simulink model "navigator"  (R2021a)
settings: Solver=FixedStepAuto  StartTime=0.0  StopTime=10.0  FixedStep=0.05  RelTol=1e-3
undefined symbols (not defined in the file): CONSTANTS_RADIUS_OF_EARTH, GF_ACTION, GF_MAX_HOR_DIST, GF_MAX_VER_DIST
(part 2 of 3)

== stateflow chart navigator/Navigator ==
  state navigator
    state COMMAND_SUB [parallel]
      settings: executionOrder=1
      state CMD_DO_GO_AROUND [parallel]
        en:
        % 临时给输出赋值，后续删除
        position_sp_triplet = pos_sp_triplet_input;
        mission_result.timestamp = uint64(getSimulationTime);
        %
        settings: executionOrder=1
        state not_running
        state running
          en:
          %publish_vehicle_command_ack(cmd, vehicle_command_s::VEHICLE_CMD_RESULT_ACCEPTED);
        (default) -> navigator.COMMAND_SUB.CMD_DO_GO_AROUND.not_running
        navigator.COMMAND_SUB.CMD_DO_GO_AROUND.not_running -> navigator.COMMAND_SUB.CMD_DO_GO_AROUND.running : [vehicle_command.command == PX4_VEHICLE_COMMAND.VEHICLE_CMD_DO_GO_AROUND]
        navigator.COMMAND_SUB.CMD_DO_GO_AROUND.running -> navigator.COMMAND_SUB.CMD_DO_GO_AROUND.not_running : [vehicle_command.command ~= PX4_VEHICLE_COMMAND.VEHICLE_CMD_DO_GO_AROUND]
      state CMD_DO_REPOSITION [parallel]
        settings: executionOrder=2
        state not_running
        state running
          en:
          get_reposition_setpoint;
        (default) -> navigator.COMMAND_SUB.CMD_DO_REPOSITION.not_running
        navigator.COMMAND_SUB.CMD_DO_REPOSITION.not_running -> navigator.COMMAND_SUB.CMD_DO_REPOSITION.running : [vehicle_command.command == PX4_VEHICLE_COMMAND.VEHICLE_CMD_DO_REPOSITION ]
        navigator.COMMAND_SUB.CMD_DO_REPOSITION.running -> navigator.COMMAND_SUB.CMD_DO_REPOSITION.not_running : [vehicle_command.command ~= PX4_VEHICLE_COMMAND.VEHICLE_CMD_DO_REPOSITION]
      state CMD_NAV_TAKEOFF [parallel]
        settings: executionOrder=3
        state not_running
        state running
          en:
          % 前一航点
          if ((home_position.timestamp > 0) && home_position.valid_alt && home_position.valid_hpos && home_position.valid_lpos)
          takeoff_triplet_.previous.valid = true;
          takeoff_triplet_.previous.timestamp = uint64(getSimulationTime);
          else
          takeoff_triplet_.previous.valid = false;
          end
          takeoff_triplet_.previous.lat = global_position.lat;
          takeoff_triplet_.previous.lon = global_position.lon;
          takeoff_triplet_.previous.alt = global_position.alt;
          takeoff_triplet_.previous.yaw = local_position.heading;
          % 当前航点
          takeoff_triplet_.current.valid = true;
          takeoff_triplet_.current.timestamp = uint64(getSimulationTime);
          takeoff_triplet_.current.type = uint8(PX4_POSITION_SETPOINT.SETPOINT_TYPE_TAKEOFF);
          if isfinite(vehicle_command.param5) && isfinite(vehicle_command.param6)
          takeoff_triplet_.current.lat = vehicle_command.param5;
          takeoff_triplet_.current.lon = vehicle_command.param6;
          else
          takeoff_triplet_.current.lat = global_position.lat;
          takeoff_triplet_.current.lon = global_position.lon;
          end
          takeoff_triplet_.current.alt = vehicle_command.param7;
          if ((home_position.timestamp > 0) && home_position.valid_alt && home_position.valid_hpos && home_position.valid_lpos)
          takeoff_triplet_.current.yaw = vehicle_command.param4;
          else
          takeoff_triplet_.current.yaw = local_position.heading;
          end
          takeoff_triplet_.current.loiter_radius = NAV_LOITER_RAD;
          takeoff_triplet_.current.loiter_direction = int8(1);
          % 下一航点
          takeoff_triplet_.next.valid = false;
        (default) -> navigator.COMMAND_SUB.CMD_NAV_TAKEOFF.not_running
        navigator.COMMAND_SUB.CMD_NAV_TAKEOFF.not_running -> navigator.COMMAND_SUB.CMD_NAV_TAKEOFF.running : [vehicle_command.command == PX4_VEHICLE_COMMAND.VEHICLE_CMD_NAV_TAKEOFF]
        navigator.COMMAND_SUB.CMD_NAV_TAKEOFF.running -> navigator.COMMAND_SUB.CMD_NAV_TAKEOFF.not_running : [vehicle_command.command ~= PX4_VEHICLE_COMMAND.VEHICLE_CMD_NAV_TAKEOFF]
      state CMD_DO_CHANGE_SPEED [parallel]
        settings: executionOrder=4
        state not_running
        state running
          en,du:
          if (vehicle_command.param2 > eps)
          % 速度指令有效
          if (vehicle_status.vehicle_type == PX4_VEHICLE_STATUS.VEHICLE_TYPE_ROTARY_WING)
          mission_cruising_speed_mc_ = vehicle_command.param2;
          else
          mission_cruising_speed_fw_ = vehicle_command.param2;
          end
          else
          % 速度指令无效
          if (vehicle_status.vehicle_type == PX4_VEHICLE_STATUS.VEHICLE_TYPE_ROTARY_WING)
          mission_cruising_speed_mc_ = single(-1);
          else
          mission_cruising_speed_fw_ = single(-1);
          end
          % 设置油门指令
          if (vehicle_command.param3 > eps)
          mission_throttle_ = vehicle_command.param3 / 100;
          else
          mission_throttle_ = single(nan);
          end
          end
          % TO DO: publish_vehicle_command_ack
        (default) -> navigator.COMMAND_SUB.CMD_DO_CHANGE_SPEED.not_running
        navigator.COMMAND_SUB.CMD_DO_CHANGE_SPEED.not_running -> navigator.COMMAND_SUB.CMD_DO_CHANGE_SPEED.running : [vehicle_command.command==PX4_VEHICLE_COMMAND.VEHICLE_CMD_DO_CHANGE_SPEED]
        navigator.COMMAND_SUB.CMD_DO_CHANGE_SPEED.running -> navigator.COMMAND_SUB.CMD_DO_CHANGE_SPEED.not_running : [vehicle_command.command~=PX4_VEHICLE_COMMAND.VEHICLE_CMD_DO_CHANGE_SPEED]
    state TRAFFIC [parallel]
      settings: executionOrder=2
    state GEOFENCE_CHECK [parallel]
      settings: executionOrder=3
    state SWITCH_NAV_STATE [parallel]
      en,du:
      switch uint8(vehicle_status.nav_state)
      case uint8(PX4_VEHICLE_STATUS.NAVIGATION_STATE_AUTO_MISSION)
      navigation_mode_ = NAVIGATION_MODE.mission;
      case uint8(PX4_VEHICLE_STATUS.NAVIGATION_STATE_AUTO_LOITER)
      navigation_mode_ == NAVIGATION_MODE.loiter;
      case uint8(PX4_VEHICLE_STATUS.NAVIGATION_STATE_AUTO_TAKEOFF)
      navigation_mode_ == NAVIGATION_MODE.takeoff;
      case uint8(PX4_VEHICLE_STATUS.NAVIGATION_STATE_AUTO_LAND)
      navigation_mode_ == NAVIGATION_MODE.land;
      case uint8(PX4_VEHICLE_STATUS.NAVIGATION_STATE_AUTO_LANDENGFAIL)
      navigation_mode_ == NAVIGATION_MODE.engineFailure;
      case uint8(PX4_VEHICLE_STATUS.NAVIGATION_STATE_AUTO_LANDGPSFAIL)
      navigation_mode_ == NAVIGATION_MODE.gpsFailure;
      case uint8(PX4_VEHICLE_STATUS.NAVIGATION_STATE_AUTO_RTL)
      switch RTL_TYPE
      case {int32(PX4_RTL_TYPE.LAND), int32(PX4_RTL_TYPE.CLOSEST)}
      case int32(PX4_RTL_TYPE.MISSION)
      otherwise
      navigation_mode_ = NAVIGATION_MODE.rtl;
      end
      otherwise
      navigation_mode_ = NAVIGATION_MODE.rtl;
      end
      % 记录当前导航状态
      previous_nav_state = vehicle_status.nav_state;
      settings: executionOrder=4
    state NAV_STATE_ACTION [parallel]
      settings: executionOrder=5
      state MISSION [parallel]
        settings: executionOrder=1
        state not_running
        state running
          en:
        (default) -> navigator.NAV_STATE_ACTION.MISSION.not_running
        navigator.NAV_STATE_ACTION.MISSION.not_running -> navigator.NAV_STATE_ACTION.MISSION.running : [navigation_mode_ == NAVIGATION_MODE.mission]
        navigator.NAV_STATE_ACTION.MISSION.running -> navigator.NAV_STATE_ACTION.MISSION.not_running : [navigation_mode_ ~= NAVIGATION_MODE.mission]
      state RTL [parallel]
        settings: executionOrder=2
        state not_running
          en,du:
          rtl_state = PX4_RTL_STATE.NONE;
          find_RTL_destination;
        state running
          en:
          % TO DO: output RTL message, home / mission / safe point
          % 垂起旋翼阶段取消mission方式的降落，因为此处已经不是mission模式了
          deny_mission_landing_ = vehicle_status.is_vtol && (vehicle_status.vehicle_type == PX4_VEHICLE_STATUS.VEHICLE_TYPE_ROTARY_WING);
          get_rtl_alt_and_rad;
          print_des_type;
          state RTL_STATE_CLIMB
            en:
            rtl_state = PX4_RTL_STATE.CLIMB;
            climb_and_return_done_ = false;
            can_loiter_at_sp_ = false;
            % 在当前位置爬升至指定高度
            if (vehicle_status.vehicle_type == PX4_VEHICLE_STATUS.VEHICLE_TYPE_ROTARY_WING)
            % 如果多旋翼则直接爬升到给定高度
            mission_item_.nav_cmd = uint16(PX4_NAVIGATION_CMD.NAV_CMD_WAYPOINT);
            else
            %如果是固定翼，则盘旋上升到给定高度
            mission_item_.nav_cmd = uint16(PX4_NAVIGATION_CMD.NAV_CMD_LOITER_TO_ALT);
            end
            mission_item_.lat = global_position.lat;
            mission_item_.lon = global_position.lon;
            mission_item_.altitude = rtl_alt;
            mission_item_.altitude_is_relative = false;
            mission_item_.yaw = local_position.heading;
            mission_item_.acceptance_radius = navigator.get_acceptance_radius;
            mission_item_.time_inside = single(0);
            mission_item_.autocontinue = true;
            mission_item_.origin =uint8(PX4_MISSION_ORIGIN.ONBOARD);
            sprintf("RTL: climb to %f m (%f m above destination) \t", double(rtl_alt), double(rtl_alt - destination.alt))
            % mavlink_log_info(_navigator->get_mavlink_log_pub(), "RTL: climb to %d m (%d m above destination)\t",(int)ceilf(_rtl_alt), (int)ceilf(_rtl_alt - _destination.alt));
            % Reset all reached flags
            waypoint_position_reached_ = false;
            waypoint_yaw_reached_ = false;
            time_wp_reached_ = uint64(0);
            % TO DO: issue_command
            % 更新当前航点
            mission_item_ = NAV_STATE_ACTION.mission_apply_limitation(mission_item_);
            NAV_STATE_ACTION.mission_item_to_position_setpoint(mission_item_);
            pos_sp_triplet_updated_ = true;
          state RTL_STATE_RETURN
            en:
            rtl_state = PX4_RTL_STATE.RETURN;
            climb_and_return_done_ = false;
            can_loiter_at_sp_ = false;
            % 返航至目标航点
            mission_item_.nav_cmd = uint16(PX4_NAVIGATION_CMD.NAV_CMD_WAYPOINT);
            mission_item_.lat = destination.lat;
            mission_item_.lon = destination.lon;
            mission_item_.altitude = rtl_alt;
            mission_item_.altitude_is_relative = false;
            destination_dist = navigator.get_distance_2_next_waypoint(destination.lat, destination.lon, global_position.lat, global_position.lon);
            if (destination_dist < RTL_MIN_DIST)
            % 如果离着陆点很近，则采用着陆的航向
            mission_item_.yaw = destination.yaw;
            else
            % 否则机头指向着陆点
            mission_item_.yaw = navigator.get_bearing_2_next_waypoint(global_position.lat, global_position.lon, destination.lat, destination.lon);
            end
            mission_item_.acceptance_radius = navigator.get_acceptance_radius;
            mission_item_.time_inside = single(0);
            mission_item_.autocontinue = true;
            mission_item_.origin = uint8(PX4_MISSION_ORIGIN.ONBOARD);
            sprintf("RTL: return at %f m (%f m above destination) \t", double(mission_item_.altitude), double(mission_item_.altitude - destination.alt))
            % Reset all reached flags
            waypoint_position_reached_ = false;
            waypoint_yaw_reached_ = false;
            time_wp_reached_ = uint64(0);
            % TO DO: issue_command
            % 更新当前航点
            mission_item_ = NAV_STATE_ACTION.mission_apply_limitation(mission_item_);
            NAV_STATE_ACTION.mission_item_to_position_setpoint(mission_item_);
            pos_sp_triplet_updated_ = true;
          state RTL_STATE_DESCEND
            en:
            rtl_state = PX4_RTL_STATE.DESCEND;
            climb_and_return_done_ = true;
            can_loiter_at_sp_ = false;
            % 下降至指定高度
            mission_item_.nav_cmd = uint16(PX4_NAVIGATION_CMD.NAV_CMD_LOITER_TO_ALT);
            mission_item_.lat = destination.lat;
            mission_item_.lon = destination.lon;
            mission_item_.altitude = min([destination.alt + RTL_DESCEND_ALT, global_position.alt, rtl_alt]);
            mission_item_.altitude_is_relative = false;
            % Except for vtol which might be still off here and should point towards this location.
            d_current = navigator.get_distance_2_next_waypoint(global_position.lat, global_position.lon, mission_item_.lat, mission_item_.lon);
            if (vehicle_status.is_vtol && (d_current > navigator.get_acceptance_radius))
            mission_item_.yaw = navigator.get_bearing_2_next_waypoint(global_position.lat, global_position.lon, mission_item_.lat, mission_item_.lon);
            else
            mission_item_.yaw = destination.yaw;
            end
            if (vehicle_status.is_vtol)
            mission_item_.loiter_radius = rtl_loiter_rad;
            end
            mission_item_.acceptance_radius = navigator.get_acceptance_radius;
            mission_item_.time_inside = single(0);
            mission_item_.autocontinue = true;
            mission_item_.origin = uint8(PX4_MISSION_ORIGIN.ONBOARD);
            % Disable previous setpoint to prevent drift.
            position_sp_triplet.previous.valid = false;
            sprintf("RTL: descend to %f m (%f m above destination) \t", double(mission_item_.altitude), double(mission_item_.altitude - destination.alt))
            % Reset all reached flags
            waypoint_position_reached_ = false;
            waypoint_yaw_reached_ = false;
            time_wp_reached_ = uint64(0);
            % TO DO: issue_command
            % 更新当前航点
            mission_item_ = NAV_STATE_ACTION.mission_apply_limitation(mission_item_);
            NAV_STATE_ACTION.mission_item_to_position_setpoint(mission_item_);
            pos_sp_triplet_updated_ = true;
          state RTL_STATE_LOITER
            en:
            rtl_state = PX4_RTL_STATE.LOITER;
            climb_and_return_done_ = true;
            can_loiter_at_sp_ = true;
            % Don't change altitude.
            mission_item_.lat = destination.lat;
            mission_item_.lon = destination.lon;
            mission_item_.altitude = min([destination.alt + RTL_DESCEND_ALT, global_position.alt, rtl_alt]);
            mission_item_.altitude_is_relative = false;
            mission_item_.yaw = destination.yaw;
            mission_item_.loiter_radius = NAV_LOITER_RAD;
            mission_item_.acceptance_radius = navigator.get_acceptance_radius;
            mission_item_.time_inside = max(RTL_LAND_DELAY, single(0.0));
            mission_item_.autocontinue = (RTL_LAND_DELAY > eps);
            mission_item_.origin = uint8(PX4_MISSION_ORIGIN.ONBOARD);
            if (RTL_LAND_DELAY > eps)
            mission_item_.nav_cmd = uint16(PX4_NAVIGATION_CMD.NAV_CMD_LOITER_TIME_LIMIT)
            sprintf("RTL: loiter %f. \t", double(mission_item_.time_inside));
            %mavlink_log_info(_navigator->get_mavlink_log_pub(), "RTL: loiter %.1fs\t", (double)get_time_inside(_mission_item));
            %events::send<float>(events::ID("rtl_loiter"), events::Log::Info, "RTL: loiter {1:.1}s", get_time_inside(_mission_item));
            else
            mission_item_.nav_cmd = uint16(PX4_NAVIGATION_CMD.NAV_CMD_LOITER_UNLIMITED);
            sprintf("RTL: completed, loitering. \t")
            %mavlink_log_info(_navigator->get_mavlink_log_pub(), "RTL: completed, loitering\t");
            %events::send(events::ID("rtl_completed_loiter"), events::Log::Info, "RTL: completed, loitering");
            end
            % Reset all reached flags
            waypoint_position_reached_ = false;
            waypoint_yaw_reached_ = false;
            time_wp_reached_ = uint64(0);
            % TO DO: issue_command
            % 更新当前航点
            mission_item_ = NAV_STATE_ACTION.mission_apply_limitation(mission_item_);
            NAV_STATE_ACTION.mission_item_to_position_setpoint(mission_item_);
            pos_sp_triplet_updated_ = true;
          state RTL_STATE_LAND
            en:
            rtl_state = PX4_RTL_STATE.LANDING;
            climb_and_return_done_ = true;
            can_loiter_at_sp_ = false;
            % Land at destination.
            mission_item_.nav_cmd = uint16(PX4_NAVIGATION_CMD.NAV_CMD_LAND);
            mission_item_.lat = destination.lat;
            mission_item_.lon = destination.lon;
            mission_item_.yaw = destination.yaw;
            mission_item_.altitude = destination.alt;
            mission_item_.altitude_is_relative = false;
            mission_item_.acceptance_radius = navigator.get_acceptance_radius;
            mission_item_.time_inside = single(0);
            mission_item_.autocontinue = true;
            mission_item_.origin = uint8(PX4_MISSION_ORIGIN.ONBOARD);
            %mission_item_.land_precision = RTL_PLD_MD;
            %if (mission_item_.land_precision == 1)
            %_navigator->get_precland()->set_mode(PrecLandMode::Opportunistic);
            %_navigator->get_precland()->on_activation();
            %elseif (mission_item_.land_precision == 2)
            %_navigator->get_precland()->set_mode(PrecLandMode::Required);
            %_navigator->get_precland()->on_activation();
            %end
            sprintf("RTL: land at destination")
            %mavlink_log_info(_navigator->get_mavlink_log_pub(), "RTL: land at destination\t");
            % %events::send(events::ID("rtl_land_at_destination"), events::Log::Info, "RTL: land at destination");
            % Reset all reached flags
            waypoint_position_reached_ = false;
            waypoint_yaw_reached_ = false;
            time_wp_reached_ = uint64(0);
            % TO DO: issue_command
            % 更新当前航点
            mission_item_ = NAV_STATE_ACTION.mission_apply_limitation(mission_item_);
            NAV_STATE_ACTION.mission_item_to_position_setpoint(mission_item_);
            pos_sp_triplet_updated_ = true;
          state RTL_MOVE_TO_LAND_HOVER_VTOL
            en:
            rtl_state = PX4_RTL_STATE.MOVE_TO_LAND_HOVER_VTOL;
            climb_and_return_done_ = true;
            can_loiter_at_sp_ = false;
            %
            mission_item_.nav_cmd = uint16(PX4_NAVIGATION_CMD.NAV_CMD_WAYPOINT);
            mission_item_.lat = destination.lat;
            mission_item_.lon = destination.lon;
            mission_item_.altitude = min([destination.alt + RTL_DESCEND_ALT, global_position.alt, rtl_alt]);
            mission_item_.altitude_is_relative = false;
            mission_item_.yaw = navigator.get_bearing_2_next_waypoint(global_position.lat, global_position.lon, mission_item_.lat, mission_item_.lon);
            mission_item_.acceptance_radius = navigator.get_acceptance_radius;
            mission_item_.origin = uint8(PX4_MISSION_ORIGIN.ONBOARD);
            % Reset all reached flags
            waypoint_position_reached_ = false;
            waypoint_yaw_reached_ = false;
            time_wp_reached_ = uint64(0);
            % TO DO: issue_command
            % 更新当前航点
            mission_item_ = NAV_STATE_ACTION.mission_apply_limitation(mission_item_);
            NAV_STATE_ACTION.mission_item_to_position_setpoint(mission_item_);
            pos_sp_triplet_updated_ = true;
          state RTL_STATE_TRANSITION_TO_MC
            en:
            rtl_state = PX4_RTL_STATE.TRANSITION_TO_MC;
            climb_and_return_done_ = true;
            can_loiter_at_sp_ = false;
            % 设置固定翼切换到旋翼的过渡点
            mission_item_.nav_cmd = uint16(PX4_NAVIGATION_CMD.NAV_CMD_DO_VTOL_TRANSITION);
            % params 是union联合体
            mission_item_.time_inside = single(PX4_VTOL_VEHICLE_STATUS.VEHICLE_VTOL_STATE_MC);
            mission_item_.acceptance_radius = single(0.0);
            mission_item_.yaw = local_position.heading;
            mission_item_.autocontinue = true;
            % Reset all reached flags
            waypoint_position_reached_ = false;
            waypoint_yaw_reached_ = false;
            time_wp_reached_ = uint64(0);
            % TO DO: issue_command
            % 更新当前航点
            mission_item_ = NAV_STATE_ACTION.mission_apply_limitation(mission_item_);
            NAV_STATE_ACTION.mission_item_to_position_setpoint(mission_item_);
            pos_sp_triplet_updated_ = true;
          state RTL_STATE_HEAD_TO_CENTER
            en:
            rtl_state = PX4_RTL_STATE.HEAD_TO_CENTER;
            climb_and_return_done_ = true;
            can_loiter_at_sp_ = false;
            %
            mission_item_.nav_cmd = uint16(PX4_NAVIGATION_CMD.NAV_CMD_WAYPOINT);
            mission_item_.lat = destination.lat;
            mission_item_.lon = destination.lon;
            mission_item_.altitude = min([destination.alt + RTL_DESCEND_ALT, global_position.alt, rtl_alt]);
            mission_item_.altitude_is_relative = false;
            mission_item_.yaw = navigator.get_bearing_2_next_waypoint(global_position.lat, global_position.lon, mission_item_.lat, mission_item_.lon);
            mission_item_.acceptance_radius = navigator.get_acceptance_radius;
            mission_item_.time_inside = single(0);
            mission_item_.autocontinue = true;
            mission_item_.origin = uint8(PX4_MISSION_ORIGIN.ONBOARD);
            % Disable previous setpoint to prevent drift.
            position_sp_triplet.previous.valid = false;
            % Reset all reached flags
            waypoint_position_reached_ = false;
            waypoint_yaw_reached_ = false;
            time_wp_reached_ = uint64(0);
            % TO DO: issue_command
            % 更新当前航点
            mission_item_ = NAV_STATE_ACTION.mission_apply_limitation(mission_item_);
            NAV_STATE_ACTION.mission_item_to_position_setpoint(mission_item_);
            pos_sp_triplet_updated_ = true;
          state RTL_STATE_LANDED
            en:
            rtl_state = PX4_RTL_STATE.LANDED
            climb_and_return_done_ = true;
            can_loiter_at_sp_ = false;
            %
            NAV_STATE_ACTION.set_idle_item;
            rtl_alt_min_ = false;
            % Reset all reached flags
            waypoint_position_reached_ = false;
            waypoint_yaw_reached_ = false;
            time_wp_reached_ = uint64(0);
            % TO DO: issue_command
            % 更新当前航点
            mission_item_ = NAV_STATE_ACTION.mission_apply_limitation(mission_item_);
            NAV_STATE_ACTION.mission_item_to_position_setpoint(mission_item_);
            pos_sp_triplet_updated_ = true;
          (default) -> RTL_STATE_DESCEND [order 2] : % 如果rtl降落点类型为MISSION_LANDING，并且飞行器处于正在降落的过程中
              | [destination.type == PX4_RTL_DESTINATION_TYPE.MISSION_LANDING && ...
              | mission_landing_in_progress_]
          (default) -> RTL_STATE_CLIMB [order 3] : % 如果飞行器的高度低于预设的降落高度
              | [global_position.alt < ((destination.alt + RTL_RETURN_ALT) || ...
              | rtl_alt_min_)]
          (default) -> RTL_STATE_RETURN [order 4]
          RTL_STATE_CLIMB -> RTL_STATE_RETURN : [NAV_STATE_ACTION.is_mission_item_reached(mission_item_)]
          RTL_STATE_RETURN -> (junction 800) : [NAV_STATE_ACTION.is_mission_item_reached(mission_item_)]
          (junction 800) -> RTL_STATE_DESCEND [order 1] : [(RTL_LAND_DELAY < -0.01 || RTL_LAND_DELAY > 0.01) || ...
              | (vehicle_status.is_vtol && vehicle_status.vehicle_type == PX4_VEHICLE_STATUS.VEHICLE_TYPE_FIXED_WING)]
          (junction 800) -> (junction 801) [order 2]
          RTL_STATE_DESCEND -> (junction 802) : [NAV_STATE_ACTION.is_mission_item_reached(mission_item_)]
          (junction 802) -> (junction 801) [order 3]
          (junction 802) -> (junction 803) [order 2] : [vehicle_status.is_vtol && ...
              | vehicle_status.vehicle_type == PX4_VEHICLE_STATUS.VEHICLE_TYPE_FIXED_WING]
          (junction 801) -> (junction 805)
          (junction 802) -> RTL_STATE_LOITER [order 1] : [RTL_LAND_DELAY < -0.01 || RTL_LAND_DELAY > 0.01]
          (junction 803) -> RTL_STATE_HEAD_TO_CENTER
          RTL_STATE_LOITER -> (junction 805) : [NAV_STATE_ACTION.is_mission_item_reached(mission_item_)]
          (junction 805) -> (junction 804)
          (junction 804) -> RTL_STATE_LAND
          RTL_STATE_TRANSITION_TO_MC -> RTL_MOVE_TO_LAND_HOVER_VTOL : [NAV_STATE_ACTION.is_mission_item_reached(mission_item_)]
          RTL_MOVE_TO_LAND_HOVER_VTOL -> RTL_STATE_LAND : [NAV_STATE_ACTION.is_mission_item_reached(mission_item_)]
          RTL_STATE_HEAD_TO_CENTER -> RTL_STATE_TRANSITION_TO_MC : [NAV_STATE_ACTION.is_mission_item_reached(mission_item_)]
          RTL_STATE_LAND -> RTL_STATE_LANDED : [NAV_STATE_ACTION.is_mission_item_reached(mission_item_)]
          (default) -> RTL_STATE_LANDED [order 1] : % 飞行器已经着陆
              | [land_detected.landed]
        (default) -> navigator.NAV_STATE_ACTION.RTL.not_running
        navigator.NAV_STATE_ACTION.RTL.not_running -> navigator.NAV_STATE_ACTION.RTL.running : [navigation_mode_ == NAVIGATION_MODE.rtl]
        navigator.NAV_STATE_ACTION.RTL.running -> navigator.NAV_STATE_ACTION.RTL.not_running : [navigation_mode_ ~= NAVIGATION_MODE.rtl]
      state LOITER [parallel]
        settings: executionOrder=3
        state not_running
          en,du:
          loiter_pos_set = false;
        state on_activation_active
          state reposition
            en:
            % rep的数据在navigator_main.cpp中处理
            position_sp_triplet.current.velocity_valid = false;
            position_sp_triplet.previous.yaw = local_position.heading;
            position_sp_triplet.previous.lat = global_position.lat;
            position_sp_triplet.previous.lon = global_position.lon;
            position_sp_triplet.previous.alt = global_position.alt
            % 当前航路点用rep中表示
            position_sp_triplet.current = reposition_triplet_.current;
            % 下一个航路点无效
            position_sp_triplet.next.valid = false;
            % 更新标志位
            can_loiter_at_sp_ = (position_sp_triplet.current.type==PX4_POSITION_SETPOINT.SETPOINT_TYPE_LOITER);
            pos_sp_triplet_updated_ = true;
            % 设置reposition无效
            reposition_triplet_.current.valid = false;
          state disarmed
            en:
            loiter_pos_set = false;
          state set_loiter_pos
            en:
            loiter_pos_set = true;
            % 若已着陆并上锁
            if ((vehicle_status.arming_state ~= PX4_VEHICLE_STATUS.ARMING_STATE_ARMED) && land_detected.landed)
            position_sp_triplet.current.type = uint8(PX4_POSITION_SETPOINT.SETPOINT_TYPE_IDLE);
            can_loiter_at_sp_ = false;
            pos_sp_triplet_updated_ = true;
            loiter_pos_set = false;
            else
            mission_item_.nav_cmd = uint16(PX4_NAVIGATION_CMD.NAV_CMD_LOITER_UNLIMITED);
            % set current mission item to loiter
            if (can_loiter_at_sp_ && position_sp_triplet.current.valid)
            % 在当前的目标航点盘旋
            mission_item_.lat = pos_sp_triplet_input.current.lat;
            mission_item_.lon = pos_sp_triplet_input.current.lon;
            mission_item_.altitude = pos_sp_triplet_input.current.alt;
            else
            % 在当前位置盘旋
            mission_item_.lat = global_position.lat;
            mission_item_.lon = global_position.lon;
            mission_item_.altitude = global_position.alt;
            % （最小起飞高度 > 0 && item中的高度低于最小起飞的绝对高度），防止loiter高度在地面以下
            if (MIS_LTRMIN_ALT > 0) && (mission_item_.altitude < home_position.alt + MIS_LTRMIN_ALT)
            mission_item_.altitude = home_position.alt + MIS_LTRMIN_ALT;
            end
            end
            end
            mission_item_.altitude_is_relative = false;
            mission_item_.yaw = single(nan);
            mission_item_.loiter_radius = NAV_LOITER_RAD;
            mission_item_.acceptance_radius = navigator.get_acceptance_radius;
            mission_item_.time_inside = single(0.0);
            mission_item_.autocontinue = false;
            mission_item_.origin = uint8(PX4_MISSION_ORIGIN.ONBOARD);
            % convert mission item to current setpoint
            position_sp_triplet.previous.valid = false;
            % 当前航点
            position_sp_triplet.current.velocity_valid = false;
            position_sp_triplet.previous.velocity_valid = false;
            mission_item_ = NAV_STATE_ACTION.mission_apply_limitation(mission_item_);
            NAV_STATE_ACTION.mission_item_to_position_setpoint(mission_item_);
            %下一航点
            position_sp_triplet.next.valid = false;
            % 更新标志位
            can_loiter_at_sp_ = (position_sp_triplet.current.type==PX4_POSITION_SETPOINT.SETPOINT_TYPE_LOITER);
            pos_sp_triplet_updated_ = true;
          navigator.NAV_STATE_ACTION.LOITER.on_activation_active -> reposition [order 1] : [reposition_triplet_.current.valid]
          (default) -> (junction 846)
          reposition -> disarmed : [vehicle_status.arming_state ~= PX4_VEHICLE_STATUS.ARMING_STATE_ARMED]
          (junction 846) -> reposition [order 1] : [reposition_triplet_.current.valid]
          (junction 846) -> (junction 847) [order 2]
          (junction 847) -> set_loiter_pos
        (default) -> navigator.NAV_STATE_ACTION.LOITER.not_running
        navigator.NAV_STATE_ACTION.LOITER.not_running -> navigator.NAV_STATE_ACTION.LOITER.on_activation_active : [navigation_mode_ == NAVIGATION_MODE.loiter]
        navigator.NAV_STATE_ACTION.LOITER.on_activation_active -> navigator.NAV_STATE_ACTION.LOITER.not_running [order 1] : [navigation_mode_ ~= NAVIGATION_MODE.loiter]
      state TAKEOFF [parallel]
        settings: executionOrder=4
        state not_running
        state on_activation_active
          state set_takeoff_pos
            en:
            set_takeoff_position;
          state item_reached
            en:
            mission_result.finished = true;
            mission_result_updated_ = true;
            % 设置loiter项，让控制器不搞起飞那套的逻辑
            % set loiter item so position controllers stop doing takeoff logic
            NAV_STATE_ACTION.set_loiter_item(-1);
            mission_item_ = NAV_STATE_ACTION.mission_apply_limitation(mission_item_);
            NAV_STATE_ACTION.mission_item_to_position_setpoint(mission_item_);
            pos_sp_triplet_updated_ = true;
          navigator.NAV_STATE_ACTION.TAKEOFF.on_activation_active -> (junction 863) [order 1]
          (junction 863) -> (junction 864) [order 2]
          (junction 863) -> set_takeoff_pos [order 1] : [takeoff_triplet_.current.valid]
          (junction 864) -> item_reached : [~mission_result.finished && ...
              | NAV_STATE_ACTION.is_mission_item_reached(mission_item_)]
          (default) -> set_takeoff_pos
        (default) -> navigator.NAV_STATE_ACTION.TAKEOFF.not_running
        navigator.NAV_STATE_ACTION.TAKEOFF.not_running -> navigator.NAV_STATE_ACTION.TAKEOFF.on_activation_active : [navigation_mode_==NAVIGATION_MODE.takeoff]
        navigator.NAV_STATE_ACTION.TAKEOFF.on_activation_active -> navigator.NAV_STATE_ACTION.TAKEOFF.not_running [order 1] : [navigation_mode_~=NAVIGATION_MODE.takeoff]
      state ENGINE_FAILURE [parallel]
        settings: executionOrder=5
        state not_running
          en,du:
          % ef_state: engine failure state
          ef_state = PX4_EFSTATE.EF_STATE_NONE;
        state on_activation_active
          state activation
            en:
            ef_state = PX4_EFSTATE.EF_STATE_NONE;
            advance_ef;
            set_ef_item;
          state active
            en:
            advance_ef;
            set_ef_item;
          navigator.NAV_STATE_ACTION.ENGINE_FAILURE.on_activation_active -> navigator.NAV_STATE_ACTION.ENGINE_FAILURE.on_activation_active.active [order 1] : [NAV_STATE_ACTION.is_mission_item_reached(mission_item_)]
          (default) -> navigator.NAV_STATE_ACTION.ENGINE_FAILURE.on_activation_active.activation
        (default) -> navigator.NAV_STATE_ACTION.ENGINE_FAILURE.not_running
        navigator.NAV_STATE_ACTION.ENGINE_FAILURE.not_running -> navigator.NAV_STATE_ACTION.ENGINE_FAILURE.on_activation_active : [navigation_mode_ == NAVIGATION_MODE.engineFailure]
        navigator.NAV_STATE_ACTION.ENGINE_FAILURE.on_activation_active -> navigator.NAV_STATE_ACTION.ENGINE_FAILURE.not_running [order 1] : [navigation_mode_ ~= NAVIGATION_MODE.engineFailure]
      state GPS_FAILURE [parallel]
        settings: executionOrder=6
        state not_running
          en,du:
          % 仅在setpoint移动时重置GPS_FAILURE状态
          if (~can_loiter_at_sp_)
          gpsf_state = PX4_GPSFSTATE.GPSF_STATE_NONE;
          end
        state on_activation_active
          state activation
            en:
            gpsf_state = PX4_GPSFSTATE.GPSF_STATE_NONE;
            timestamp_activation = uint64(getSimulationTime);
            advance_gpsf;
            set_gpsf_item;
          state active
            en:
            switch (gpsf_state)
            case PX4_GPSFSTATE.GPSF_STATE_LOITER
            % 在这种情况下，不会运行位置控制器；所以navigator在这里发布姿态的setpoint
            % att_sp.timestamp = uint64(getSimulationTime);
            % att_sp.roll_body = single(deg2rad(NAV_GPSF_R));
            % att_sp.pitch_body = single(deg2rad(NAV_GPSF_P));
            % att_sp.thrust_body(1) = NAV_GPSF_TR;
            % att_sp.q_d = euler_to_quat(att_sp.roll_body, att_sp.pitch_body, 0);
            % TO DO: publish att_sp
            %
            % measure time
            if (NAV_GPSF_LT > eps) && ((uint64(getSimulationTime) - timestamp_activation) > NAV_GPSF_LT)
            sprintf("GPS not recovered, switching to next failure state. \n")
            advance_gpsf;
            end
            case PX4_GPSFSTATE.GPSF_STATE_TERMINATE
            set_gpsf_item;
            advance_gpsf;
            otherwise
            end
          navigator.NAV_STATE_ACTION.GPS_FAILURE.on_activation_active -> navigator.NAV_STATE_ACTION.GPS_FAILURE.on_activation_active.active [order 1]
          (default) -> navigator.NAV_STATE_ACTION.GPS_FAILURE.on_activation_active.activation
        (default) -> navigator.NAV_STATE_ACTION.GPS_FAILURE.not_running
        navigator.NAV_STATE_ACTION.GPS_FAILURE.not_running -> navigator.NAV_STATE_ACTION.GPS_FAILURE.on_activation_active : [navigation_mode_ == NAVIGATION_MODE.gpsFailure]
        navigator.NAV_STATE_ACTION.GPS_FAILURE.on_activation_active -> navigator.NAV_STATE_ACTION.GPS_FAILURE.not_running [order 1] : [navigation_mode_ ~= NAVIGATION_MODE.gpsFailure]
      state LAND [parallel]
        settings: executionOrder=7
        state not_running
        state on_activation_active
          state activation
            en:
            set_land_item(true);
            mission_result.finished = false;
            mission_result_updated_ = true;
            % reset_mission_item_reached
            waypoint_position_reached_ = false;
            waypoint_yaw_reached_ = false;
            time_wp_reached_ = uint64(0);
            % convert mission item to current setpoint
            % 当前航点
            mission_item_ = NAV_STATE_ACTION.mission_apply_limitation(mission_item_);
            NAV_STATE_ACTION.mission_item_to_position_setpoint(mission_item_);
            % 前一航点
            position_sp_triplet.previous.valid = false;
            % 下一航点
            position_sp_triplet.next.valid = false;
            % 置标志位
            can_loiter_at_sp_ = false;
            pos_sp_triplet_updated_ = true;
          state active
            en:
            % for VTOL update landing location during back transition
            position_sp_triplet.current.lat = global_position.lat;
            position_sp_triplet.current.lon = global_position.lon;
            pos_sp_triplet_updated_ = true;
          state Landed
            en:
            mission_result.finished = true;
            mission_result_updated_ = true;
            NAV_STATE_ACTION.set_idle_item;
            NAV_STATE_ACTION.mission_item_to_position_setpoint(mission_item_);
            pos_sp_triplet_updated_ = true;
          navigator.NAV_STATE_ACTION.LAND.on_activation_active -> (junction 906) [order 1]
          (default) -> navigator.NAV_STATE_ACTION.LAND.on_activation_active.activation
          (junction 906) -> (junction 907) [order 2]
          (junction 906) -> navigator.NAV_STATE_ACTION.LAND.on_activation_active.active [order 1] : % 飞机是vtol机型，并且处于过渡模式
              | [vehicle_status.is_vtol && vehicle_status.in_transition_mode]
          (junction 907) -> Landed : % 飞机已经着陆
              | [land_detected.landed]
        (default) -> navigator.NAV_STATE_ACTION.LAND.not_running
        navigator.NAV_STATE_ACTION.LAND.not_running -> navigator.NAV_STATE_ACTION.LAND.on_activation_active : [navigation_mode_ == NAVIGATION_MODE.land]
        navigator.NAV_STATE_ACTION.LAND.on_activation_active -> navigator.NAV_STATE_ACTION.LAND.not_running [order 1] : [navigation_mode_ ~= NAVIGATION_MODE.land]
  data: previous_nav_state local uint8 size=1 =uint8(3); destination_check_time local uint64 size=1 =uint64(0); rtl_state local Enum: PX4_RTL_STATE size=1; rtl_loiter_rad local single size=1; rtl_alt local single size=1; destination local Bus: px4_rtl_position; destination_check_time local uint64 size=1 =uint64(0); destination_dist local single; d_current local single size=1; rtl_state local Enum: PX4_RTL_STATE size=1; rtl_loiter_rad local single size=1; rtl_alt local single size=1; destination local Bus: px4_rtl_position size=1; deny_mission_landing_ local boolean size=1 =false; mission_landing_in_progress_ local boolean size=1 =false; climb_and_return_done_ local boolean size=1 =false; loiter_pos_set local boolean size=1 =false; ef_state local Enum: PX4_EFSTATE size=1; item_in function_input; itme_out function_output; item function_input; isreached function_output; item function_input; gpsf_state local Enum: PX4_GPSFSTATE size=1; timestamp_activation local uint64 size=1; at_current_location function_input; item function_output; min_clearance function_input; min_clearance function_input; item function_output; waypoint_position_reached_ local boolean size=1 =false; waypoint_yaw_reached_ local boolean size=1 =false; time_wp_reached_ local uint64 size=1 =uint64(0); mission_item_yaw function_input; out function_output; speed function_output; phi function_input; theta function_input; psi function_input; q0 function_output; q1 function_output; q2 function_output; q3 function_output; lat_now function_input; lon_now function_input; lat_next function_input; lon_next function_input; dist function_output; radius function_output single; out function_output single; out function_output; lat_now function_input; lon_now function_input; lat_next function_input; lon_next function_input; bearing function_output; acc_radius function_output single; time function_output; item function_input; item_altitude_is_relative function_input; alt function_output single; item_altitude function_input; vehicle_command input Bus: px4_vehicle_command size=1; global_position input Bus: px4_vehicle_global_position size=1; local_position input Bus: px4_vehicle_local_position size=1; vehicle_status input Bus: px4_vehicle_status size=1; RTL_RETURN_ALT parameter size=1; RTL_CONE_ANG parameter size=1; RTL_LOITER_RAD parameter size=1; NAV_ACC_RAD parameter size=1; pos_sp_triplet_updated_ local boolean size=1; land_detected input Bus: px4_vehicle_land_detected size=1; pos_sp_triplet_input input Bus: px4_position_setpoint_triplet size=1; home_position input Bus: px4_home_position size=1; NAV_LOITER_RAD parameter size=1; pos_ctrl_status input Bus: px4_position_controller_status size=1; position_sp_triplet output Bus: px4_position_setpoint_triplet size=1; MIS_LTRMIN_ALT parameter size=1; mission_throttle_ local single size=1 =single(nan); mission_cruising_speed_mc_ local single size=1 =single(-1.0); mission_cruising_speed_fw_ local single size=1 =single(-1.0); reposition_triplet_ local Bus: px4_position_setpoint_triplet size=1; takeoff_triplet_ local Bus: px4_position_setpoint_triplet size=1; MIS_TAKEOFF_ALT parameter size=1; mission_result output Bus: px4_mission_result size=1; NAV_GPSF_R parameter size=1; NAV_GPSF_P parameter size=1; NAV_GPSF_TR parameter size=1; NAV_GPSF_LT parameter size=1; CONSTANTS_RADIUS_OF_EARTH parameter single size=1; RTL_MIN_DIST parameter single size=1; rtl_alt_min_ local boolean size=1 =false; RTL_DESCEND_ALT parameter size=1; RTL_LAND_DELAY parameter size=1; RTL_PLD_MD parameter size=1; RTL_TYPE parameter size=1; VT_B_DEC_MSS parameter size=1; VT_B_REV_DEL parameter size=1; MIS_YAW_ERR parameter size=1; MIS_YAW_TMT parameter size=1; NAV_FW_ALTL_RAD parameter size=1; NAV_FW_ALT_RAD parameter size=1; NAV_MC_ALT_RAD parameter size=1; GF_ACTION parameter size=1; MPC_JERK_AUTO parameter size=1; MPC_ACC_HOR parameter size=1; navigation_mode_ local Enum: NAVIGATION_MODE size=1; mission_item_ local Bus: px4_navigator_mission_item size=1; mission_result_updated_ local boolean size=1 =false; can_loiter_at_sp_ local boolean size=1 =false
  function get_reposition_setpoint:
    | function get_reposition_setpoint
    | 
    | %% 判断reposition是否在禁飞区内
    | if (GF_ACTION ~= PX4_GEOFENCE_RESULT.GF_ACTION_NONE &&  GF_ACTION ~= PX4_GEOFENCE_RESULT.GF_ACTION_WARN)
    |     %mavlink_log_critical(&_mavlink_log_pub, "Reposition is outside geofence\t");
    |     %events::send(events::ID("navigator_reposition_outside_geofence"), {events::Log::Error, events::LogInternal::Info},
    |     %"Reposition is outside geofence");
    |     return;
    | end
    | 
    | 
    | %% 初始化上个航点
    | reposition_triplet_.previous.valid = true;
    | reposition_triplet_.previous.timestamp = uint64(getSimulationTime);
    | reposition_triplet_.previous.lat = global_position.lat;
    | reposition_triplet_.previous.lon = global_position.lon;
    | reposition_triplet_.previous.alt = global_position.alt;
    | reposition_triplet_.previous.yaw = local_position.heading;
    | 
    | %% 初始化当前航点
    | reposition_triplet_.current.valid = true;
    | reposition_triplet_.current.timestamp = uint64(getSimulationTime);
    | reposition_triplet_.current.loiter_radius = NAV_LOITER_RAD;
    | reposition_triplet_.current.loiter_direction = int8(1);
    | reposition_triplet_.current.type = uint8(PX4_POSITION_SETPOINT.SETPOINT_TYPE_LOITER);
    | 
    | % 如果没有速度参数，使用默认值
    | if (vehicle_command.param1 <= 0 || ~isfinite(vehicle_command.param1))
    |     reposition_triplet_.current.cruising_speed = navigator.get_cruising_speed();
    | else
    |     reposition_triplet_.current.cruising_speed = vehicle_command.param1;
    | end
    | % 油门
    | reposition_triplet_.current.cruising_throttle = navigator.get_cruising_throttle;
    | % 提前量
    | reposition_triplet_.current.acceptance_radius = navigator.get_acceptance_radius;
    | % 偏航角
    | if isfinite(vehicle_command.param4)
    |     reposition_triplet_.current.yaw = vehicle_command.param4;
    |     reposition_triplet_.current.yaw_valid = true;
    | else
    |     reposition_triplet_.current.yaw = single(nan);
    |     reposition_triplet_.current.yaw_valid = false;
    | end
    | % 经纬高
    | if isfinite(vehicle_command.param5) && isfinite(vehicle_command.param6)
    |     % 经纬度有效
    |     reposition_triplet_.current.lat = vehicle_command.param5;
    |     reposition_triplet_.current.lon = vehicle_command.param6;
    |     if isfinite(vehicle_command.param7)
    |         reposition_triplet_.current.alt = vehicle_command.param7;
    |     else
    |         reposition_triplet_.current.alt = global_position.alt;
    |     end
    | elseif vehicle_command.param7
    |     % 经纬度无效，高度有效
    |     reposition_triplet_.current.lat = pos_sp_triplet_input.current.lat;
    |     reposition_triplet_.current.lon = pos_sp_triplet_input.current.lon;
    |     reposition_triplet_.current.alt = vehicle_command.param7;
    | else
    |     % 经纬高均无效
    |     reposition_triplet_.current.alt = global_position.alt;
    |     
    |     if vehicle_status.vehicle_type == PX4_VEHICLE_STATUS.VEHICLE_TYPE_ROTARY_WING && pos_sp_triplet_input.current.type ~= uint8(PX4_POSITION_SETPOINT.SETPOINT_TYPE_TAKEOFF)
    |         % 多旋翼计算刹车距离，确定悬停位置
    |         course_over_ground = atan2(local_position.vy, local_position.vx);
    |         velocity_hor_abs = sqrt(local_position.vx^2 + local_position.vy^2);
    |         multirotor_braking_distance = velocity_hor_abs * (velocity_hor_abs / (2 * MPC_ACC_HOR) + (0.6 * MPC_JERK_AUTO) / MPC_JERK_AUTO);
    |         
    |         [reposition_triplet_.current.lat, reposition_triplet_.current.lon] = waypoint_from_heading_and_distance(global_position.lat, global_position.lon,...
    |                                                                                 course_over_ground, multirotor_braking_distance);
    |         reposition_triplet_.current.yaw = local_position.heading;
    |         reposition_triplet_.current.yaw_valid = true;
    |     else
    |         % 固定翼使用当前位置进行盘旋
    |         reposition_triplet_.current.lat = global_position.lat;
    |         reposition_triplet_.current.lon = global_position.lon;
    |     end
    | end
    | 
    | %% 初始化下个航点
    | reposition_triplet_.next.valid = false;
    | 
    | end
  function find_RTL_destination:
    | function find_RTL_destination
    | 
    | destination = initial;
    | 
    | 
    | % if (getSimulationTime - destination_check_time) >= 1 && (home_position.timestamp > 0) && home_position.valid_alt && home_position.valid_hpos && home_position.valid_lpos
    | %     destination_check_time = getSimulationTime;
    | %     
    | %     % set destination to home per default, then check if other valid landing spot is closer
    | %     destination.lat = home_position.lat;
    | %     destination.lon = home_position.lon;
    | %     destination.alt = home_position.alt;
    | %     destination.yaw = home_position.yaw;
    | %     destination.safe_point_index = uint8(0);
    | %     destination.type = uint8(PX4_RTL_DESTINATION_TYPE.HOME);
    | %     
    | %     lon_scale = cos(deg2rad(global_position.lat));
    | %     
    | %     % get distance to home position
    | %     dlat = home_position.lat - global_position.lat;
    | %     dlon = home_position.lon - global_position.lon;
    | %     min_dist_squared = coord_dist_sq(dlat, dlon, lon_scale);
    | %     
    | %     % consider the mission landing if not RTL_HOME type set
    | %     if (RTL_TYPE ~= PX4_RTL_TYPE.HOME) && land_start_available_
    | %         if vehicle_status.is_vtol && (vehicle_status.vehicle_type == PX4_VEHICLE_STATUS.VEHICLE_TYPE_ROTARY_WING)
    | %             mission_landing_lat = landing_lat_;
    | %             mission_landing_lon = landing_lon_;
    | %             mission_landing_alt = landing_alt_;
    | %             destination_type = uint8(PX4_RTL_DESTINATION_TYPE.HOME);
    | %         else
    | %             mission_landing_lat = landing_start_lat_;
    | %             mission_landing_lon = landing_start_lon_;
    | %             mission_landing_alt = landing_start_alt_;
    | %             destination_type = uint8(PX4_RTL_DESTINATION_TYPE.MISSION_LANDING);
    | %         end
    | %         
    | %         % compare home position to landing position to decide which is closer
    | %         dlat = mission_landing_lat - global_position.lat;
    | %         dlon = mission_landing_lon - global_position.lon;
    | %         dist_squared = coord_dist_sq(dlat, dlon, lon_scale);
    | %         
    | %         if (dist_squared < min_dist_squared) || (RTL_TYPE ~= PX4_RTL_TYPE.CLOSEST)
    | %             min_dist_squared = dist_squared;
    | %             destination.lat = mission_landing_lat;
    | %             destination.lon = mission_landing_lon;
    | %             destination.alt = mission_landing_alt;
    | %             destination.type = destination_type;
    | %         end
    | %     end
    | %     
    | %     % 涉及到航点读取，未做
    | % end
    | 
    | end
    | 
    | 
    | %% 
    | function out = initial
    | out.lat = home_position.lat;
    | out.lon = home_position.lon;
    | out.alt = home_position.alt;
    | out.yaw = home_position.yaw;
    | out.safe_point_index = uint8(0);
    | out.type = uint8(PX4_RTL_DESTINATION_TYPE.HOME);
    | end
    | 
    | 
    | %% 
    | function out = coord_dist_sq(lat_diff,lon_diff,lon_scale)
    | 
    | lon_diff_scaled = lon_scale * wrap(lon_diff, -180, 180);
    | out = lat_diff * lat_diff + lon_diff_scaled * lon_diff_scaled;
    | 
    | end
  function get_rtl_alt_and_rad:
    |      function get_rtl_alt_and_rad
    | 
    | % 默认盘旋半径
    | % RTL_LOITER_RAD = 1;
    | % RTL_CONE_ANG = 1;
    | rtl_loiter_rad = RTL_LOITER_RAD;
    | 
    | % 根据处于旋翼阶段还是固定翼阶段，返回rtl高度
    | if vehicle_status.vehicle_type == PX4_VEHICLE_STATUS.VEHICLE_TYPE_ROTARY_WING
    |     rtl_alt = calculate_return_alt_from_cone_half_angle(RTL_CONE_ANG);
    | else
    |     rtl_alt = max([global_position.alt, destination.alt, home_position.alt + RTL_RETURN_ALT]);
    | end
    | 
    | end
    | 
    | %% 旋翼飞机或旋翼阶段飞机的rtl高度
    | function alt = calculate_return_alt_from_cone_half_angle(cone_half_angle_deg)
    | 
    | % horizontal distance to destination
    | % 计算飞机到降落点的水平距离
    | destination_dist = get_distance_to_next_waypoint(destination.lat, destination.lon, global_position.lat, global_position.lon);
    | 
    | % minium rtl altitude to use when outside of horizontal acceptance radius of target position.
    | % We choose the minimum height to be two times the distance from the land position in order to
    | % avoid the vehicle touching the ground while still moving horizontally.
    | % 在目标位置的水平接受半径外使用的rtl高度。我们选择最小高度的距离是距离土地位置的两倍,以避免车辆在地面移动时触碰地面。
    | return_altitude_min_outside_acceptance_rad_amsl = destination.alt + 2.0 * get_acceptance_radius;
    | 
    | return_altitude_amsl = destination.alt + RTL_RETURN_ALT;
    | 
    | if (destination_dist <= get_acceptance_radius)
    |     return_altitude_amsl = destination.alt + 2.0 * destination_dist;   
    | else
    |     if (cone_half_angle_deg > 0) && (destination_dist <= RTL_MIN_DIST)
    |         
    |         % constrain cone half angle to meaningful values. All other cases are already handled above.
    |         cone_half_angle_rad = deg2rad(constrain(cone_half_angle_deg, 1, 89));
    |         
    |         % minimum altitude we need in order to be within the user defined cone
    |         cone_intersection_altitude_amsl = destination_dist / tan(cone_half_angle_rad) + destination.alt;
    |         
    |         return_altitude_amsl = min(cone_intersection_altitude_amsl, return_altitude_amsl);
    |     end
    |     
    |     return_altitude_amsl = max(return_altitude_amsl, return_altitude_min_outside_acceptance_rad_amsl);
    | end
    | 
    | alt = max(return_altitude_amsl, global_position.alt);
    | 
    | end
  function print_des_type:
    | function print_des_type
    | 
    | % 打印rtl目的点的类型
    | % output the correct message, depending on where the RTL destination is
    | switch (uint8(destination.type))
    |     case uint8(PX4_RTL_DESTINATION_TYPE.HOME)
    |         sprintf("RTL: landing at home position.");
    |         
    |     case uint8(PX4_RTL_DESTINATION_TYPE.MISSION_LANDING)
    |         sprintf("RTL: landing at mission landing.");
    |         
    |     case uint8(PX4_RTL_DESTINATION_TYPE.SAFE_POINT)
    |         sprintf("RTL: landing at safe landing point.");
    | end
    |         
    | end
  function set_takeoff_position:
    | function set_takeoff_position
    | 
    | %% 确定默认的起飞高度
    | % 如果home点有效，起飞高度为home点的海平面高度加上起飞的最小高度
    | if ((home_position.timestamp > 0) && home_position.valid_alt && home_position.valid_hpos && home_position.valid_lpos)
    |     min_abs_altitude = global_position.alt + MIS_TAKEOFF_ALT;
    | else
    |     min_abs_altitude = MIS_TAKEOFF_ALT;
    | end
    | 
    | %% 如果用户设置了起飞高度
    | % takeoff_triplet_是在navigator_main.cpp中通过获取cmd参数得到的lat,lon,alt
    | if (takeoff_triplet_.current.valid && isfinite(takeoff_triplet_.current.alt) && ...
    |         (home_position.timestamp > 0) && home_position.valid_alt && home_position.valid_hpos && home_position.valid_lpos)
    |     % 使用用户设置的起飞高度
    |     abs_altitude = takeoff_triplet_.current.alt;
    |     if (abs_altitude < min_abs_altitude)
    |         abs_altitude = min_abs_altitude;
    |     end
    |     sprintf("Using minimum takeoff altitude: %f m", double(MIS_TAKEOFF_ALT))
    |     % mavlink_log_critical
    | else
    |     abs_altitude = min_abs_altitude;
    |     sprintf("Using minimum takeoff altitude: %f m", double(MIS_TAKEOFF_ALT))
    |     % mavlink_log_info
    | end
    | 
    | if (abs_altitude < global_position.alt)
    |     % If the suggestion is lower than our current alt, let's not go down
    |     abs_altitude = global_position.alt;
    |     sprintf("Already higher than takeoff altitude")
    | end
    | 
    | set_takeoff_item(abs_altitude);
    | 
    | mission_result.finished = false;
    | mission_result_updated_ = true;
    | waypoint_position_reached_ = false;
    | waypoint_yaw_reached_ = false;
    | time_wp_reached_ = uint64(0);
    | 
    | % convert mission item to current setpoint
    | mission_item_ = mission_apply_limitation(mission_item_);
    | mission_item_to_position_setpoint(mission_item_);
    | position_sp_triplet.current.yaw_valid = true;
    | 
    | if takeoff_triplet_.current.valid
    |     position_sp_triplet.current.lat = takeoff_triplet_.current.lat;
    |     position_sp_triplet.current.lon = takeoff_triplet_.current.lon;
    |     position_sp_triplet.current.yaw = IsFinite(takeoff_triplet_.current.yaw, position_sp_triplet.current.yaw);
    |     takeoff_triplet_.current.valid = false;
    | end
    | 
    | % 前一航点
    | position_sp_triplet.previous.valid = false;
    | % 下一航点
    | position_sp_triplet.next.valid = false;
    | 
    | % 置标志位
    | if (isfinite(position_sp_triplet.current.lat) && isfinite(position_sp_triplet.current.lon))
    |     can_loiter_at_sp_ = true;
    | else
    |     can_loiter_at_sp_ = false;
    | end
    | 
    | pos_sp_triplet_updated_ = true;
    | 
    | end
    | 
    | %% 设置takeoff_item
    | function set_takeoff_item(alt)
    | 
    | mission_item_.nav_cmd = uint16(PX4_NAVIGATION_CMD.NAV_CMD_TAKEOFF);
    | mission_item_.lat = global_position.lat;
    | mission_item_.lon = global_position.lon;
    | mission_item_.yaw = local_position.heading;
    | mission_item_.altitude = alt;
    | mission_item_.altitude_is_relative = false;
    | mission_item_.loiter_radius = NAV_LOITER_RAD;
    | mission_item_.autocontinue = false;
    | mission_item_.origin = uint8(PX4_MISSION_ORIGIN.ONBOARD);
    | 
    | end
  function advance_ef:
    | function advance_ef
    | 
    | switch (ef_state)
    |     
    |     case PX4_EFSTATE.EF_STATE_NONE
    |         sprintf("Engine failure. Loitering down. \n")
    |         % mavlink_log_emergency
    |         ef_state = PX4_EFSTATE.EF_STATE_LOITERDOWN;
    |         
    |     otherwise
    |         
    | end
    | 
    | end
  function set_ef_item:
    | function set_ef_item
    | 
    | % 由于engine failure，将当前的setpoint设置为上一个setpoint，飞机也不能loiter
    | position_sp_triplet.previous = position_sp_triplet.current;
    | can_loiter_at_sp_ = false;
    | 
    | switch (ef_state)
    |     
    |     case PX4_EFSTATE.EF_STATE_LOITERDOWN
    |         % 在飞机的当前位置创建一个mission_item
    |         mission_item_.lat = global_position.lat;
    |         mission_item_.lon = global_position.lon;
    |         mission_item_.altitude_is_relative = false;
    |         mission_item_.altitude = single(home_position.alt - 1000.0); % setting altitude to a very low value
    |         mission_item_.yaw = single(nan);
    |         mission_item_.loiter_radius = NAV_LOITER_RAD;
    |         mission_item_.nav_cmd = uint16(PX4_NAVIGATION_CMD.NAV_CMD_LOITER_UNLIMITED);
    |         mission_item_.acceptance_radius = navigator.get_acceptance_radius;
    |         mission_item_.autocontinue = true;
    |         mission_item_.origin = uint8(PX4_MISSION_ORIGIN.ONBOARD);
    |         can_loiter_at_sp_ = true;
    |         
    |     otherwise
    |         
    | end
    | 
    | % reset_mission_item_reached
    | waypoint_position_reached_ = false;
    | waypoint_yaw_reached_ = false;
    | time_wp_reached_ = uint64(0);
    | 
    | % convert mission item to current position setpoint and make it valid
    | mission_item_ = NAV_STATE_ACTION.mission_apply_limitation(mission_item_);
    | NAV_STATE_ACTION.mission_item_to_position_setpoint(mission_item_);
    | position_sp_triplet.next.valid = false;
    | 
    | pos_sp_triplet_updated_ = true;
    | 
    | end
  function itme_out = mission_apply_limitation(item_in):
    | function itme_out = mission_apply_limitation(item_in)
    | 
    | % Limit altitude
    | itme_out = item_in;
    | 
    | if (land_detected.alt_max > 0.0)
    |     % absolute altitude
    |     altitude_abs = selection(item_in.altitude_is_relative, eps, item_in.altitude + home_position.alt, item_in.altitude);
    |     
    |     % limit altitude to maximum allowed altitude
    |     if ((land_detected.alt_max + home_position.alt) < altitude_abs)
    |         itme_out.altitude = selection(item_in.altitude_is_relative, 0, land_detected.alt_max, land_detected.alt_max + home_position.alt);
    |     end
    |     
    | end
    | 
    | end
  function set_idle_item:
    | function set_idle_item
    | 
    | mission_item_.nav_cmd = uint16(PX4_NAVIGATION_CMD.NAV_CMD_IDLE);
    | mission_item_.lat = home_position.lat;
    | mission_item_.lon = home_position.lon;
    | mission_item_.time_inside = single(0.0);
    | mission_item_.acceptance_radius = get_acceptance_radius;
    | mission_item_.loiter_radius = NAV_LOITER_RAD;
    | mission_item_.yaw = single(nan);
    | mission_item_.altitude = home_position.alt;
    | mission_item_.origin = uint8(PX4_MISSION_ORIGIN.ONBOARD);
    | mission_item_.altitude_is_relative = false;
    | mission_item_.autocontinue = true;
    | 
    | end
  function mission_item_to_position_setpoint(item):
    | % Convert a mission item to a position setpoint
    | function mission_item_to_position_setpoint(item)
    | 
    | % TO DO: don't change the setpoint for non-position items
    | % if (!item_contains_position(item)) {
    | % 		return false;
    | % 	}
    | 
    | position_sp_triplet.current.timestamp = uint64(getSimulationTime);
    | position_sp_triplet.current.valid = true;
    | 
    | %% 纬度、经度、高度、航向、航向有效性
    | position_sp_triplet.current.lat = item.lat;
    | position_sp_triplet.current.lon = item.lon;
    | position_sp_triplet.current.alt = get_absolute_altitude_for_item(item.altitude_is_relative, item.altitude);
    | position_sp_triplet.current.yaw = item.yaw;
    | position_sp_triplet.current.yaw_valid = isfinite(item.yaw);
    | 
    | %% 盘旋半径、盘旋方向、提前量
    | position_sp_triplet.current.loiter_radius = selection(abs(item.loiter_radius), 0.001, abs(item.loiter_radius), NAV_LOITER_RAD);
    | position_sp_triplet.current.loiter_direction = int8(sign(item.loiter_radius));
    | if isfinite(item.acceptance_radius) && (item.acceptance_radius > 0.0)
    |     position_sp_triplet.current.acceptance_radius = item.acceptance_radius;
    | else
    |     position_sp_triplet.current.acceptance_radius = NAV_ACC_RAD;
    | end
    | 
    | %% 巡航速度、巡航油门
    | position_sp_triplet.current.cruising_speed = navigator.get_cruising_speed;
    | position_sp_triplet.current.cruising_throttle = selection(mission_throttle_, eps, mission_throttle_, single(nan));
    | 
    | 
    | %% 设置mission item.cmd
    | switch item.nav_cmd
    |     
    |     case PX4_NAVIGATION_CMD.NAV_CMD_IDLE
    |         position_sp_triplet.current.type = uint8(PX4_POSITION_SETPOINT.SETPOINT_TYPE_IDLE);
    |         
    |     case PX4_NAVIGATION_CMD.NAV_CMD_TAKEOFF
    |         % if already flying (armed and !landed) treat TAKEOFF like regular POSITION
    |         if ((vehicle_status.arming_state == PX4_VEHICLE_STATUS.ARMING_STATE_ARMED) && ~land_detected.landed && ~land_detected.maybe_landed)
    |             position_sp_triplet.current.type = uint8(PX4_POSITION_SETPOINT.SETPOINT_TYPE_POSITION);
    |         else
    |             position_sp_triplet.current.type = uint8(PX4_POSITION_SETPOINT.SETPOINT_TYPE_TAKEOFF);
    |         end
    |         
    |     case PX4_NAVIGATION_CMD.NAV_CMD_VTOL_TAKEOFF
    |         position_sp_triplet.current.type = uint8(PX4_POSITION_SETPOINT.SETPOINT_TYPE_TAKEOFF);
    |         
    |     case {PX4_NAVIGATION_CMD.NAV_CMD_LAND, PX4_NAVIGATION_CMD.NAV_CMD_VTOL_LAND} 
    |         position_sp_triplet.current.type = uint8(PX4_POSITION_SETPOINT.SETPOINT_TYPE_LAND);
    |         
    |     case PX4_NAVIGATION_CMD.NAV_CMD_LOITER_TO_ALT
    |         
    |         position_sp_triplet.current.type = uint8(PX4_POSITION_SETPOINT.SETPOINT_TYPE_LOITER);
    |         
    |         % MIS_LTRMIN_ALT：这是飞机需要遵守的最低高度，目的是排除地面效应；设置为-1，如果不应该有最小的loiter高度
    |         if (MIS_LTRMIN_ALT > 0.0)
    |             position_sp_triplet.current.alt = max(global_position.alt, home_position.alt + MIS_LTRMIN_ALT);
    |         else
    |             position_sp_triplet.current.alt = global_position.alt;
    |         end
    | 
    |     case {PX4_NAVIGATION_CMD.NAV_CMD_LOITER_TIME_LIMIT, PX4_NAVIGATION_CMD.NAV_CMD_LOITER_UNLIMITED}
    |         position_sp_triplet.current.type = uint8(PX4_POSITION_SETPOINT.SETPOINT_TYPE_LOITER);
    |         
    |     otherwise
    |         position_sp_triplet.current.type = uint8(PX4_POSITION_SETPOINT.SETPOINT_TYPE_POSITION);
    |         
    | end
    | 
    | % position_sp_triplet.current.disable_weather_vane = true;
    | 
    | % %%%%%%%%%%%%%%%%%%%%%%%%%%%%%%%%%%%%%%%%%%%%
    | % position_sp_triplet.current.vx = single(nan);
    | % position_sp_triplet.current.vy = single(nan);
    | % position_sp_triplet.current.vz = single(nan);
    | % position_sp_triplet.current.velocity_valid = false;
    | % position_sp_triplet.current.velocity_frame = uint8(0);
    | % position_sp_triplet.current.alt_valid = true;
    | % 
    | % position_sp_triplet.current.yawspeed = single(nan);
    | % position_sp_triplet.current.yawspeed_valid = false;
    | % position_sp_triplet.current.landing_gear = int8(0);
    | % 
    | 
    | end
  function isreached = is_mission_item_reached(item):
    | function isreached = is_mission_item_reached(item)
    | 
    | isreached = false;
    | 
    | % 处理非导航指令和非定义的航点
    | switch item.nav_cmd
    |     
    |     case uint16(PX4_NAVIGATION_CMD.NAV_CMD_DO_SET_SERVO)
    |         isreached = true;
    |         
    |     case {uint16(PX4_NAVIGATION_CMD.NAV_CMD_LAND), uint16(PX4_NAVIGATION_CMD.NAV_CMD_VTOL_LAND)}
    |         isreached = land_detected.landed;
    |         
    |     case {uint16(PX4_NAVIGATION_CMD.NAV_CMD_IDLE), uint16(PX4_NAVIGATION_CMD.NAV_CMD_LOITER_UNLIMITED)}
    |         isreached = false;
    |         
    |     case {uint16(PX4_NAVIGATION_CMD.NAV_CMD_DO_LAND_START),               uint16(PX4_NAVIGATION_CMD.NAV_CMD_DO_TRIGGER_CONTROL), ...
    |             uint16(PX4_NAVIGATION_CMD.NAV_CMD_DO_DIGICAM_CONTROL),          uint16(PX4_NAVIGATION_CMD.NAV_CMD_IMAGE_START_CAPTURE), ...
    |             uint16(PX4_NAVIGATION_CMD.NAV_CMD_IMAGE_STOP_CAPTURE),          uint16(PX4_NAVIGATION_CMD.NAV_CMD_VIDEO_START_CAPTURE), ...
    |             uint16(PX4_NAVIGATION_CMD.NAV_CMD_VIDEO_STOP_CAPTURE),          uint16(PX4_NAVIGATION_CMD.NAV_CMD_DO_CONTROL_VIDEO), ...
    |             uint16(PX4_NAVIGATION_CMD.NAV_CMD_DO_MOUNT_CONFIGURE),          uint16(PX4_NAVIGATION_CMD.NAV_CMD_DO_MOUNT_CONTROL), ...
    |             uint16(PX4_NAVIGATION_CMD.NAV_CMD_DO_GIMBAL_MANAGER_PITCHYAW),  uint16(PX4_NAVIGATION_CMD.NAV_CMD_DO_GIMBAL_MANAGER_CONFIGURE), ...
    |             uint16(PX4_NAVIGATION_CMD.NAV_CMD_DO_SET_ROI),                  uint16(PX4_NAVIGATION_CMD.NAV_CMD_DO_SET_ROI_LOCATION), ...
    |             uint16(PX4_NAVIGATION_CMD.NAV_CMD_DO_SET_ROI_WPNEXT_OFFSET),    uint16(PX4_NAVIGATION_CMD.NAV_CMD_DO_SET_ROI_NONE), ...
    |             uint16(PX4_NAVIGATION_CMD.NAV_CMD_DO_SET_CAM_TRIGG_DIST),       uint16(PX4_NAVIGATION_CMD.NAV_CMD_OBLIQUE_SURVEY), ...
    |             uint16(PX4_NAVIGATION_CMD.NAV_CMD_DO_SET_CAM_TRIGG_INTERVAL),   uint16(PX4_NAVIGATION_CMD.NAV_CMD_SET_CAMERA_MODE), ...
    |             uint16(PX4_NAVIGATION_CMD.NAV_CMD_SET_CAMERA_ZOOM),             uint16(PX4_NAVIGATION_CMD.NAV_CMD_SET_CAMERA_FOCUS)}
    |         isreached = true;
    |         
    |     case uint16(PX4_NAVIGATION_CMD.NAV_CMD_DO_VTOL_TRANSITION)
    |         if (item.time_inside == 3)
    |             isreached = (vehicle_status.vehicle_type == PX4_VEHICLE_STATUS.VEHICLE_TYPE_ROTARY_WING);
    |         elseif (item.time_inside == 4)
    |             isreached = (vehicle_status.vehicle_type == PX4_VEHICLE_STATUS.VEHICLE_TYPE_FIXED_WING);
    |         else
    |             isreached = false;
    |         end
    |         
    |     case {uint16(PX4_NAVIGATION_CMD.NAV_CMD_DO_CHANGE_SPEED), uint16(PX4_NAVIGATION_CMD.NAV_CMD_DO_SET_HOME)}
    |         isreached = true;
    | end
    | 
    | %% 如果飞机没有着陆并且还没有到达指定航点
    | if (~land_detected.landed && ~waypoint_position_reached_)
    |     
    |     % 将mission_item中的高度转换为绝对海平面高度
    |     mission_item_altitude_amsl = navigator.get_absolute_altitude_for_item(item.altitude_is_relative, item.altitude);
    |     % 计算到航点的距离
    |     [dist_xy, dist_z, dist] = get_distance_to_point_global_wgs84(item.lat, item.lon, mission_item_altitude_amsl, ...
    |         global_position.lat, global_position.lon, global_position.alt);
    |     
    |     if ((item.nav_cmd == uint16(PX4_NAVIGATION_CMD.NAV_CMD_TAKEOFF)) || (item.nav_cmd == uint16(PX4_NAVIGATION_CMD.NAV_CMD_VTOL_TAKEOFF)) && ...
    |             (vehicle_status.vehicle_type == PX4_VEHICLE_STATUS.VEHICLE_TYPE_ROTARY_WING))
    |         
    |         %% 垂起/多旋翼起飞
    |         takeoff_alt = selection(item.altitude_is_relative, eps, item.altitude, item.altitude - home_position.alt); % 起飞高度换算成对地高度
    |         altitude_acceptance_radius = get_altitude_acceptance_radius;
    |         
    |         if (takeoff_alt > 0.0) && (takeoff_alt < altitude_acceptance_radius)
    |             altitude_acceptance_radius = takeoff_alt / 2;
    |         end
    |         
    |         % 飞机的高度到达了默认提前量的一半，认为到达了航点
    |         if (global_position.alt > (mission_item_altitude_amsl - altitude_acceptance_radius))
    |             waypoint_position_reached_ = true;
    |         end
    |         
    |     elseif (vehicle_status.vehicle_type == PX4_VEHICLE_STATUS.VEHICLE_TYPE_ROVER) && (item.nav_cmd == uint16(PX4_NAVIGATION_CMD.NAV_CMD_TAKEOFF))
    |         
    |         %% 无人车的先不管
    |         
    |     elseif item.nav_cmd == uint16(PX4_NAVIGATION_CMD.NAV_CMD_TAKEOFF)
    |         
    |         %% 固定翼起飞
    |         if ((dist >= 0 && dist <= get_acceptance_radius) && (dist_z <= get_altitude_acceptance_radius))
    |             waypoint_position_reached_ = true;
    |         end
    |         
    |     elseif (vehicle_status.vehicle_type == PX4_VEHICLE_STATUS.VEHICLE_TYPE_FIXED_WING) && ...
    |             (item.nav_cmd == uint16(PX4_NAVIGATION_CMD.NAV_CMD_LOITER_UNLIMITED) || item.nav_cmd == uint16(PX4_NAVIGATION_CMD.NAV_CMD_LOITER_TIME_LIMIT))
    |         
    |         %% 固定翼按时间盘旋
    |         if ((dist >= 0.0) && (dist_xy <= (get_acceptance_radius + abs(item.loiter_radius))) && (dist_z <= get_altitude_acceptance_radius))
    |             waypoint_position_reached_ = true;
    |         end
    |         
    |     elseif item.nav_cmd == uint16(PX4_NAVIGATION_CMD.NAV_CMD_LOITER_TO_ALT)
    |         
    |         %% 固定翼盘旋到高度
    |         % nav_loiter_to_alt只有在loiter中使用任务项高度。
    |         % 第一次检查海拔基准点是任务定点（这意味着loiter还没有到达）
    |         if (abs(pos_sp_triplet_input.current.alt - mission_item_altitude_amsl) >= eps)
    |             [dist_xy1, dist_z1, dist1] = get_distance_to_point_global_wgs84(item.lat, item.lon, pos_sp_triplet_input.current.alt, ...
    |                 global_position.lat, global_position.lon, global_position.alt);
    |             
    |             if ((dist1 >= 0) && (dist_xy1 <= (get_acceptance_radius + abs(item.loiter_radius))) && (dist_z1 <= get_default_altitude_acceptance_radius))
    |                 position_sp_triplet.current.alt = mission_item_altitude_amsl;
    |                 position_sp_triplet.current.type = uint8(PX4_POSITION_SETPOINT.SETPOINT_TYPE_LOITER);
    |                 pos_sp_triplet_updated_ = true;
    |             end
    |             
    |         elseif ((dist >= 0.0) && (dist_xy <= (get_acceptance_radius + abs(item.loiter_radius))) && (dist_z <= get_altitude_acceptance_radius))
    |             waypoint_position_reached_ = true;
    |         end
    |         
    |     elseif (item.nav_cmd == uint16(PX4_NAVIGATION_CMD.NAV_CMD_CONDITION_GATE))
    |         
    |         %% item中的航点是否在飞机与当前期望航点之间
    |         
    |     elseif item.nav_cmd == uint16(PX4_NAVIGATION_CMD.NAV_CMD_DELAY)
    |         
    |         %% delay
    |         waypoint_position_reached_ = true;
    |         waypoint_yaw_reached_ = true;
    |         time_wp_reached_ = uint64(getSimulationTime);
    |         
    |     else
    |         acceptance_radius = get_acceptance_radius;
    |         if ((vehicle_status.vehicle_type == PX4_VEHICLE_STATUS.VEHICLE_TYPE_ROTARY_WING) && isfinite(item.acceptance_radius) && (item.acceptance_radius > eps))
    |             % 新的提前量
    |             acceptance_radius = item.acceptance_radius;
    |         end
    |         
    |         % for vtol back transition calculate acceptance radius based on time and ground speed
    |         if ((item.vtol_back_transition) && (vehicle_status.vehicle_type == PX4_VEHICLE_STATUS.VEHICLE_TYPE_FIXED_WING))
    |             velocity = sqrt(local_position.vx^2 + local_position.vy^2);
    |             
    |             if ((VT_B_DEC_MSS > eps) && (velocity > eps))
    |                 acceptance_radius = ((velocity / VT_B_DEC_MSS / 2) * velocity) + VT_B_REV_DEL * velocity;
    |             end
    |         end
    |         
    |         if ((dist_xy >= 0.0) && (dist_xy <= acceptance_radius) && (dist_z <= get_altitude_acceptance_radius))
    |             waypoint_position_reached_ = true;
    |         end
    |     end
    |     
    |     %% 记录航点到达的时间
    |     if (waypoint_position_reached_)
    |         time_wp_reached_ = uint64(getSimulationTime);
    |     end
    |     
    |     if (vehicle_status.vehicle_type ~= PX4_VEHICLE_STATUS.VEHICLE_TYPE_ROTARY_WING)
    |         % consider yaw reached for fixed-wing
    |         waypoint_yaw_reached_ = true;
    |     end
    |     
    | end
    | 
    | %% 检查所要求的yaw setpoint是否达到（只用于旋翼飞行）
    | if (waypoint_position_reached_ && ~waypoint_yaw_reached_)
    |     if vehicle_status.vehicle_type == PX4_VEHICLE_STATUS.VEHICLE_TYPE_ROTARY_WING && isfinite(get_yaw_acceptance(item.yaw))
    |         
    |         % 多旋翼会判断yaw是否到达
    |         yaw_error = wrap(item.yaw - local_position.heading, -pi, pi);
    |         
    |         if (abs(yaw_error) < deg2rad(MIS_YAW_ERR) || (MIS_YAW_TMT >= eps && ~item.force_heading))
    |             waypoint_yaw_reached_ = true;
    |         end
    |         
    |         % 如果航点到达了，但是在规定的时间内没有到达指定的yaw
    |         if ((~waypoint_yaw_reached_) && (item.force_heading && (MIS_YAW_TMT >= eps)) && ...
    |                 (uint64(getSimulationTime) - time_wp_reached_)/1000 >= MIS_YAW_TMT) % unit s
    |             % 设置mission失败
    |             sprintf("unable to reach heading within timeout. \n")
    |             % set_mission_failure_heading_timeout();
    |         end
    |     else
    |         % 固定翼不需要判断yaw是否到达
    |         waypoint_yaw_reachead = true;
    |     end
    | end
    | 
    | %% time是否达到
    | if (waypoint_position_reached_ && waypoint_yaw_reached_)
    |     
    |     % 如果航点到达且航向到达，那么开始判断inside_time是否到达
    |     time_inside_reached = false;
    |     
    |     if (get_time_inside(item) < eps) || ((uint64(getSimulationTime) - time_wp_reached_)/1000 >= get_time_inside(item)) % unit s
    |         % check if the MAV was long enough inside the waypoint orbit
    |         time_inside_reached = true;
    |     end
    |     
    |     %% 检查是否到达出口（只适用于固定翼飞行）
    |     exit_heading_reached = false;
    |     
    |     if (time_inside_reached)
    |         % enforce exit heading if in FW, the next wp is valid, the vehicle is currently loitering and either having force_heading set,
    |         % or if loitering to achieve altitdue at a NAV_CMD_WAYPOINT
    |         % 如果在FW中执行退出，那么下一个wp是有效的，该飞机目前正在进行loitering，要么有force_heading设置，要么是在NAV_CMD_WAYPOINT上实现altitdue
    |         enforce_exit_heading = ((vehicle_status.vehicle_type ~= PX4_VEHICLE_STATUS.VEHICLE_TYPE_ROTARY_WING) && pos_sp_triplet_input.next.valid && ...
    |             pos_sp_triplet_input.current.type == uint8(PX4_POSITION_SETPOINT.SETPOINT_TYPE_LOITER) && ...
    |             (item.force_heading || item.nav_cmd == uint16(PX4_NAVIGATION_CMD.NAV_CMD_WAYPOINT)));
    |         
    |         if (enforce_exit_heading)
    |             % check if heading for exit is reached (only applies for fixed-wing)
    |             dist_current_next = get_distance_to_next_waypoint(pos_sp_triplet_input.current.lat, pos_sp_triplet_input.current.lon, ...
    |                 pos_sp_triplet_input.next.lat, pos_sp_triplet_input.next.lon);
    |             
    |             if (dist_current_next > 1.2 * NAV_LOITER_RAD)
    |                 item.yaw = get_bearing_to_next_waypoint(global_position.lat, global_position.lon, pos_sp_triplet_input.next.lat, pos_sp_triplet_input.next.lon);
    |                 cog = atan2(local_position.vy, local_position.vx);
    |                 yaw_err = wrap(item.yaw - cog, -pi, pi);
    |             else
    |                 yaw_err = single(0.0);
    |             end
    |             
    |             if (abs(yaw_err) < deg2rad(MIS_YAW_ERR))
    |                 exit_heading_reached = true;
    |             end
    |             
    |         else
    |             exit_heading_reached = true;
    |         end
    |         
    |     end
    |     
    |     %% 设置退出飞行路线到下一个地点
    |     if (exit_heading_reached)
    |         % set exit flight course to next waypoint
    |         % 计算当前sp与下一个sp之间的距离
    |         range = get_distance_to_next_waypoint(pos_sp_triplet_input.current.lat, pos_sp_triplet_input.current.lon, ...
    |             pos_sp_triplet_input.next.lat, pos_sp_triplet_input.next.lon);
    |         
    |         % reset lat/lon of loiter waypoint so vehicle follows a tangent
    |         % 重置lat/lon的转线点，因此车辆遵循切线
    |         if (item.loiter_exit_xtrack && pos_sp_triplet_input.next.valid && isfinite(range) && ...
    |                 (item.nav_cmd == uint16(PX4_NAVIGATION_CMD.NAV_CMD_LOITER_TIME_LIMIT) || item.nav_cmd == uint16(PX4_NAVIGATION_CMD.NAV_CMD_LOITER_TO_ALT)))
    | 
    |             bearing = get_bearing_to_next_waypoint(pos_sp_triplet_input.current.lat, pos_sp_triplet_input.current.lon, pos_sp_triplet_input.next.lat, pos_sp_triplet_input.next.lon);
    |             ratio = constrain(item.loiter_radius / range, -1, 1);
    |             inner_angle = pi/2 - asin(ratio);
    |             
    |             if (pos_sp_triplet_input.current.loiter_direction > 0.0)
    |                 bearing = bearing - inner_angle;
    |             else
    |                 bearing = bearing + inner_angle;
    |             end
    |             
    |             % Replace current setpoint lat/lon with tangent coordinate
    |             [position_sp_triplet.current.lat, position_sp_triplet.current.lon] = waypoint_from_heading_and_distance(pos_sp_triplet_input.current.lat, pos_sp_triplet_input.current.lon, ...
    |                 bearing, abs(pos_sp_triplet_input.current.loiter_radius));
    |         end
    |         
    |         isreached = true;
    |         
    |     end
    | end
    | 
    | end
  function advance_gpsf:
    | function advance_gpsf
    | 
    | switch (gpsf_state)
    |     
    |     case PX4_GPSFSTATE.GPSF_STATE_NONE
    |         gpsf_state = PX4_GPSFSTATE.GPSF_STATE_LOITER;
    |         
    |     case PX4_GPSFSTATE.GPSF_STATE_LOITER
    |         gpsf_state = PX4_GPSFSTATE.GPSF_STATE_TERMINATE;
    |         
    |     case PX4_GPSFSTATE.GPSF_STATE_TERMINATE
    |         gpsf_state = PX4_GPSFSTATE.GPSF_STATE_END;
    |         
    |     otherwise
    |         
    | end
    |     
    | end
  function set_gpsf_item:
    | function set_gpsf_item
    |  
    | position_sp_triplet.previous.valid = false;
    | position_sp_triplet.current.valid = false;
    | position_sp_triplet.next.valid = false;
    | 
    | switch gpsf_state
    |     
    |     case (PX4_GPSFSTATE.GPSF_STATE_TERMINATE)
    |         
    |         mission_result.flight_termination = true;
    |         mission_result_updated_ = true;
    |         sprintf("GPS failure: request flight termination. \n")
    |         
    |     otherwise
    |         
    | end
    | 
    | pos_sp_triplet_updated_ = true;
    | 
    | end
  function set_land_item(at_current_location):
    | % set current mission item to Land
    | function set_land_item(at_current_location)
    | 
    | % VTOL transition to RW before landing
    | % 对于vtol机型，降落前需要转换为旋翼
    | % if navigator->force_vtol()
    | %     vcmd.command = NAV_CMD_DO_VTOL_TRANSITION;
    | %     vcmd.param1 = vtol_vehicle_status_s::VEHICLE_VTOL_STATE_MC;
    | %     vcmd.param2 = 0.0f;
    | %     _navigator->publish_vehicle_cmd(&vcmd);
    | % end
    | 
    | % set the land item
    | mission_item_.nav_cmd = uint16(PX4_NAVIGATION_CMD.NAV_CMD_LAND);
    | 
    | if at_current_location
    |     % use current position
    |     mission_item_.lat = double(nan); % descend at current position
    |     mission_item_.lon = double(nan);
    |     mission_item_.yaw = local_position.heading;
    | else
    |     % use home position
    |     mission_item_.lat = home_position.lat;
    |     mission_item_.lon = home_position.lon;
    |     mission_item_.yaw = home_position.yaw;
    | end
    | 
    | mission_item_.altitude = single(0.0);
    | mission_item_.altitude_is_relative = false;
    | mission_item_.loiter_radius = NAV_LOITER_RAD;
    | mission_item_.acceptance_radius = navigator.get_acceptance_radius;
    | mission_item_.time_inside = single(0.0);
    | mission_item_.autocontinue = true;
    | mission_item_.origin = uint8(PX4_MISSION_ORIGIN.ONBOARD);
    | 
    | end
  function item = set_loiter_item2(min_clearance):
    | function item = set_loiter_item2(min_clearance)
    | 
    | if land_detected.landed
    | %     item.nav_cmd = uint16(PX4_NAVIGATION_CMD.IDLE);
    |     item = set_idle_item;
    | else
    |     item.timestamp = uint64(getSimulationTime);
    |     item.instance_count = uint32(0);
    |     item.sequence_current = uint16(0);
    | 
    |     item.nav_cmd = uint16(PX4_NAVIGATION_CMD.NAV_LOITER_UNLIM);
    |     if can_loiter_at_sp_ && pos_sp_triplet_input.current.valid
    |         % 目标点经纬度
    |         item.lat = pos_sp_triplet_input.current.lat;
    |         item.lon = pos_sp_triplet_input.current.lon;
    |     else
    |         % 飞机当前经纬度
    |         item.lat = global_position.lat;
    |         item.lon = global_position.lon;
    |     end
    |     
    |     item.time_inside = single(0);
    |     item.acceptance_radius = get_acceptance_radius;
    |     item.loiter_radius = NAV_LOITER_RAD;
    |     item.yaw = single(nan);
    |     
    |     if can_loiter_at_sp_ && pos_sp_triplet_input.current.valid
    |         item.altitude = pos_sp_triplet_input.current.alt;
    |     else
    |         item.altitude = global_position.alt;
    |         if (min_clearance > 0) && (item.altitude < home_position.alt + min_clearance)
    |             item.altitude = home_position.alt + min_clearance;
    |         end
    |     end
    |     
    |     item.frame = uint8(0);
    |     item.origin = uint8(PX4_MISSION_ORIGIN.ONBOARD);
    |     item.loiter_exit_xtrack = false;
    |     item.force_heading = false;
    |     
    |     item.altitude_is_relative = false;
    |     item.autocontinue = false;
    |     item.vtol_back_transition = false;
    | end
    | 
    | end
  function set_loiter_item(min_clearance):
    | function set_loiter_item(min_clearance)
    | 
    | if land_detected.landed
    |     mission_item.nav_cmd = uint16(PX4_NAVIGATION_CMD.NAV_CMD_IDLE);
    | %     mission_item = set_idle_item;
    | else
    |     mission_item.nav_cmd = uint16(PX4_NAVIGATION_CMD.NAV_CMD_LOITER_UNLIMITED);
    |     if (can_loiter_at_sp_ && pos_sp_triplet_input.current.valid)
    |         % 目标点经纬度
    |         mission_item.lat = pos_sp_triplet_input.current.lat;
    |         mission_item.lon = pos_sp_triplet_input.current.lon;
    |         mission_item.altitude = pos_sp_triplet_input.current.alt;
    |     else
    |         % 飞机当前经纬度
    |         mission_item.lat = global_position.lat;
    |         mission_item.lon = global_position.lon;
    |         mission_item.altitude = global_position.alt;
    |         if (min_clearance > 0) && (mission_item.altitude < home_position.alt + min_clearance)
    |             mission_item.altitude = home_position.alt + min_clearance;
    |         end
    |     end
    |     
    |     mission_item.time_inside = single(0);
    |     mission_item.acceptance_radius = get_acceptance_radius;
    |     mission_item.loiter_radius = NAV_LOITER_RAD;
    |     mission_item.yaw = single(nan);
    |     
    |     mission_item.origin = uint8(PX4_MISSION_ORIGIN.ONBOARD);
    |     mission_item.altitude_is_relative = false;
    |     mission_item.autocontinue = false;
    | end
    | 
    | end
  function item = set_idle_item2:
    | function item = set_idle_item2
    | 
    | item.timestamp = uint64(getSimulationTime);
    | item.instance_count = uint32(0);
    | item.sequence_current = uint16(0);
    | item.nav_cmd = uint16(PX4_NAVIGATION_CMD.IDLE);
    | item.lat = home_position.lat;
    | item.lon = home_position.lon;
    | item.time_inside = single(0);
    | item.acceptance_radius = get_acceptance_radius;
    | item.loiter_radius = NAV_LOITER_RAD;
    | item.yaw = single(nan);
    | item.altitude = home_position.alt;
    | item.frame = uint8(0);
    | item.origin = uint8(PX4_MISSION_ORIGIN.ONBOARD);
    | item.loiter_exit_xtrack = false;
    | item.force_heading = false;
    | item.altitude_is_relative = false;
    | item.autocontinue = true;
    | item.vtol_back_transition = false;
    | 
    | end
  function out = get_yaw_acceptance(mission_item_yaw):
    | function out = get_yaw_acceptance(mission_item_yaw)
    | out = mission_item_yaw;
    | 
    | % if yaw_acceptance from position controller is NaN overwrite the mission item yaw such that
    | % the waypoint can be reached from any direction
    | if (pos_ctrl_status.timestamp > pos_sp_triplet_input.timestamp) && ~isfinite(pos_ctrl_status.yaw_acceptance)
    |     out = pos_ctrl_status.yaw_acceptance;
    | end
    | 
    | end
  function speed = get_cruising_speed:
    | function speed = get_cruising_speed
    | 
    | if vehicle_status.vehicle_type == PX4_VEHICLE_STATUS.VEHICLE_TYPE_ROTARY_WING
    |     if (navigation_mode_ == NAVIGATION_MODE.mission) && (mission_cruising_speed_mc_ > 0.0)
    |         speed = mission_cruising_speed_mc_;
    |     else
    |         speed = single(-1);
    |     end
    | else
    |     if (navigation_mode_ == NAVIGATION_MODE.mission) && (mission_cruising_speed_fw_ > 0.0)
    |         speed = mission_cruising_speed_fw_;
    |     else
    |         speed = single(-1);
    |     end
    | end
    | 
    | end
  function [q0,q1,q2,q3] = euler_to_quat(phi,theta,psi):
    | function [q0,q1,q2,q3] = euler_to_quat(phi,theta,psi)
    | [q0,q1,q2,q3] = euler2quat(phi,theta,psi);
    | end
  function dist = get_distance_2_next_waypoint(lat_now,lon_now,lat_next,lon_next):
    | function dist = get_distance_2_next_waypoint(lat_now,lon_now,lat_next,lon_next)
    |  
    | dist = get_distance_to_next_waypoint(lat_now,lon_now,lat_next,lon_next);
    | 
    | end
  function radius = get_altitude_acceptance_radius:
    | function radius = get_altitude_acceptance_radius
    | 
    | radius = get_default_altitude_acceptance_radius;
    | 
    | if vehicle_status.vehicle_type == PX4_VEHICLE_STATUS.VEHICLE_TYPE_FIXED_WING && pos_sp_triplet_input.next.type == uint8(PX4_POSITION_SETPOINT.SETPOINT_TYPE_LAND) && pos_sp_triplet_input.next.valid
    |     % Use separate (tighter) altitude acceptance for clean altitude starting point before landing
    |     radius = NAV_FW_ALTL_RAD;
    | end
    | 
    | end
  function out = get_cruising_throttle:
    | function out = get_cruising_throttle
    | 
    | if (mission_throttle_ > eps)
    |     out = mission_throttle_;
    | else
    |     out = single(nan);
    | end
    | 
    | end
  function out = get_default_altitude_acceptance_radius:
    | function out = get_default_altitude_acceptance_radius
    |  
    | if vehicle_status.vehicle_type == PX4_VEHICLE_STATUS.VEHICLE_TYPE_FIXED_WING
    |     out = NAV_FW_ALT_RAD;
    | elseif vehicle_status.vehicle_type == PX4_VEHICLE_STATUS.VEHICLE_TYPE_ROVER
    |     out = single(Inf);
    | else
    |     alt_acceptance_radius = NAV_MC_ALT_RAD;
    |     if (pos_ctrl_status.timestamp > pos_sp_triplet_input.timestamp) && (pos_ctrl_status.altitude_acceptance > alt_acceptance_radius)
    |         alt_acceptance_radius = pos_ctrl_status.altitude_acceptance;
    |     end
    |     
    |     out = alt_acceptance_radius;
    | end
    | 
    | end
  function bearing = get_bearing_2_next_waypoint(lat_now,lon_now,lat_next,lon_next):
    | function bearing = get_bearing_2_next_waypoint(lat_now,lon_now,lat_next,lon_next)
    |  
    | bearing = get_bearing_to_next_waypoint(lat_now,lon_now,lat_next,lon_next);
    | 
    | end
  function acc_radius = get_acceptance_radius:
    | function acc_radius = get_acceptance_radius
    | 
    | acc_radius = NAV_ACC_RAD;
    | 
    | % for fixed-wing, return the max of NAV_ACC_RAD and the controller acceptance radius (e.g. L1 distance)
    | if (vehicle_status.vehicle_type ~= PX4_VEHICLE_STATUS.VEHICLE_TYPE_ROTARY_WING)...
    |     && isfinite(pos_ctrl_status.acceptance_radius) && (pos_ctrl_status.timestamp ~= 0)
    | 
    |     acc_radius = max(NAV_ACC_RAD, pos_ctrl_status.acceptance_radius);
    | end
    | 
    | end
  function time = get_time_inside(item):
    | function time = get_time_inside(item)
    | 
    | time = single(0);
    | 
    | if ((item.nav_cmd == uint16(PX4_NAVIGATION_CMD.NAV_CMD_WAYPOINT) && vehicle_status.vehicle_type == PX4_VEHICLE_STATUS.VEHICLE_TYPE_ROTARY_WING) || ....
    |         item.nav_cmd == uint16(PX4_NAVIGATION_CMD.NAV_CMD_LOITER_TIME_LIMIT) || item.nav_cmd == uint16(PX4_NAVIGATION_CMD.NAV_CMD_DELAY))
    |     time = max(item.time_inside, 0);
    | end
    | 
    | end
  function alt = get_absolute_altitude_for_item(item_altitude_is_relative,item_altitude):
    | function alt = get_absolute_altitude_for_item(item_altitude_is_relative,item_altitude)
    | 
    | if item_altitude_is_relative
    |     alt = home_position.alt + item_altitude;
    | else
    |     alt = item_altitude;
    | end
    |     
    | end
